simulink model "P1_striedavy"  (R2020b)
settings: Solver=VariableStepAuto  StartTime=0.0  StopTime=10.0  RelTol=1e-3
settings Model: Creator=stank  LastModifiedBy=stank

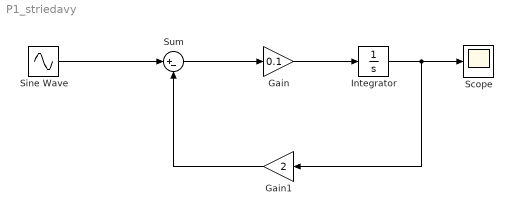
== system P1_striedavy ==
  Gain : Gain  Gain=0.1
  Gain1 : Gain  Gain=2
  Integrator : Integrator
  Scope : Scope
  Sine Wave : Sin  Amplitude=10  Frequency=50  SampleTime=0
  Sum : Sum  Inputs=|+-
  wires:
  Sine Wave/1 -> Sum/1
  Gain1/1 -> Sum/2
  Sum/1 -> Gain/1
  Gain/1 -> Integrator/1
  Integrator/1 -> Gain1/1, Scope/1
